simulink model "CBB_ccontrol_pspice_Robust"  (R2024a)
settings: Solver=VariableStepAuto  StartTime=0.0  StopTime=1  RelTol=1e-3
undefined symbols (not defined in the file): C, kr1, kr2, L, L1, M, R
libraries: pspsim x1, spsSawtoothGeneratorLib x1
settings Model: Creator=omar_  LastModifiedBy=rodol
settings DebuggingCC: UnconnectedInputMsg=warning  UnconnectedOutputMsg=warning  UnconnectedLineMsg=warning
settings ModelReferenceCC: EnableRefExpFcnMdlSchedulingChecks=on
settings RTWCC: GPUComputeCapability=3.5  DLArmComputeVersion=19.05

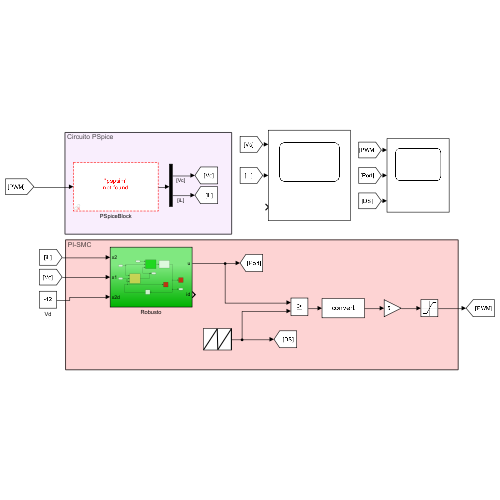
[thumbnail: Simulink's stored preview of the top-level diagram]
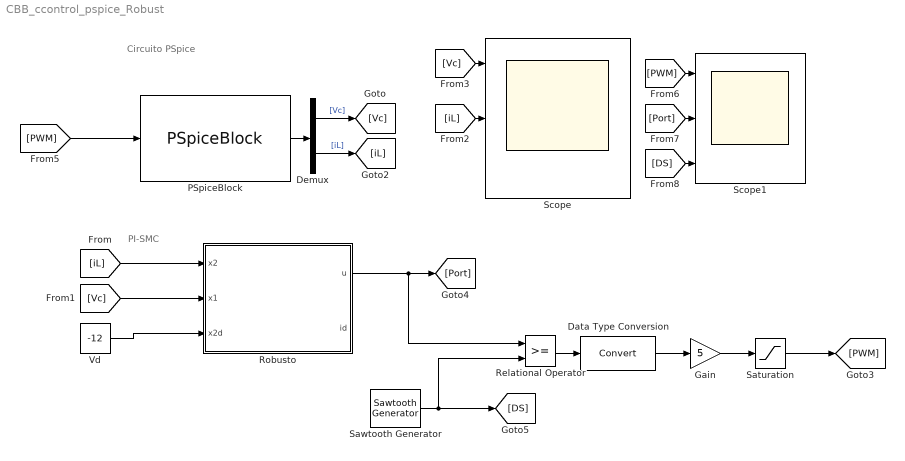
== system CBB_ccontrol_pspice_Robust ==
  note: Circuito PSpice
  note: PI-SMC
  Data Type Conversion : DataTypeConversion  SaturateOnIntegerOverflow=off  RndMeth=Floor
  Demux : Demux  Outputs=2
  Gain : Gain  Gain=5
  PSpiceBlock : pspsim/PSpiceBlock  SFunctionModules=''
      settings: SourceProductName=PSpice Block
  Relational Operator : RelationalOperator  OutDataTypeStr=boolean  RndMeth=Simplest  InputSameDT=off
  Robusto : Subsystem
  Saturation : Saturate  UpperLimit=5  LowerLimit=0
  Sawtooth Generator : spsSawtoothGeneratorLib/Sawtooth Generator  Freq=50000  Phase=0  Ts=0
  Scope : Scope  NumInputPorts=3
  Scope1 : Scope  NumInputPorts=3
  Vd : Constant  Value=-12
  wires:
  [PWM] -> PSpiceBlock/1
  [DS] -> Scope1/3
  Relational Operator/1 -> Data Type Conversion/1
  [Port] -> Scope1/2
  [iL] -> Robusto/1(x2)
  Gain/1 -> Saturation/1
  [iL] -> Scope/2
  PSpiceBlock/1 -> Demux/1
  [Vc] -> Scope/1
  Data Type Conversion/1 -> Gain/1
  Saturation/1 -> [PWM]
  Robusto/1(u) -> Relational Operator/1, [Port]
  [Vc] -> Robusto/2(x1)
  Demux/2 -> [iL]  "[iL]"
  Demux/1 -> [Vc]  "[Vc]"
  Sawtooth Generator/1 -> [DS], Relational Operator/2
  Vd/1 -> Robusto/3(x2d)
  [PWM] -> Scope1/1

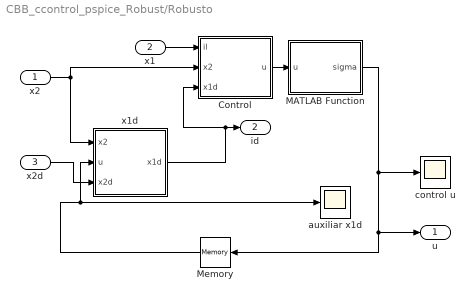
== system CBB_ccontrol_pspice_Robust/Robusto ==
  x2 : Inport
  x1 : Inport  Port=2
  x2d : Inport  Port=3
  Control : MATLAB Function  TreatAsAtomicUnit=on
  MATLAB Function : MATLAB Function  TreatAsAtomicUnit=on
  Memory : Memory
  auxiliar x1d : Scope
  control u : Scope
  x1d : MATLAB Function  TreatAsAtomicUnit=on
  u : Outport
  id : Outport  Port=2
  wires:
  x1/1 -> Control/1(il)
  x2/1 -> x1d/1(x2), Control/2(x2)
  Memory/1 -> x1d/2(u), auxiliar x1d/1
  x2d/1 -> x1d/3(x2d)
  x1d/1(x1d) -> Control/3(x1d), id/1
  MATLAB Function/1(sigma) -> Memory/1, u/1, control u/1
  Control/1(u) -> MATLAB Function/1(u)

== matlab function CBB_ccontrol_pspice_Robust/Robusto/Control ==
  data: il input; u output; x2 input; x1d input; E parameter; L parameter; kr1 parameter
function u = control(il, x2, x1d, E, L, kr1)

%error
e1 = il - x1d;

%control
%u = ( E + kr1*L*sign(e1) ) / ( x2 - E) + 1;
u = L * (kr1 * sqrt(abs(e1)) * sign(e1) + E / L) / (x2 - E) + 1;
%u = L * (kr1 * (e1) + E / L) / (x2 - E) + 1;
end

== matlab function CBB_ccontrol_pspice_Robust/Robusto/x1d ==
  data: x1d output; x2 input; u input; C parameter; R parameter; x2d input; kr2 parameter
function x1d = des(x2, u, C, R,x2d, kr2)

%error
e2 = x2 - x2d;

%Auxiliar control
x1d = C * (kr2 * sqrt(abs(e2)) * sign(e2) - (1 / (R * C)) * (e2 + x2d)) / (1 - u);

== matlab function CBB_ccontrol_pspice_Robust/Robusto/MATLAB Function ==
  data: u input; sigma output; L1 parameter; M parameter
function sigma  = fcn(u, L1, M)
    amin = (pi) / (2 * (M - L1));
    s = u;
    if s < L1
        sigma = s;
    elseif s >= L1
        %sigma = tanh(amin * (s - L1)) / amin + L1;
        sigma = (1 / amin) * tanh(amin * (s - L1)) + L1;
    else
        sigma = 0;
    end
end
